simulink model "Projekt_KUS_sim"  (R2013a)
settings: Solver=ode45  SolverMode=SingleTasking  StartTime=0.0  StopTime=1.0  RelTol=1e-3
undefined symbols (not defined in the file): B, Mn, psien, R, T, Un
settings Model: Creator=user  LastModifiedBy=Jarek
settings DataIOCC: SignalLoggingSaveFormat=ModelDataLogs
settings OptimizationCC: BlockReduction=off  BooleanDataType=off
settings DebuggingCC: SaveWithParameterizedLinksMsg=none  SignalResolutionControl=TryResolveAllWithWarning  SolverPrmCheckMsg=none  MultiTaskDSMMsg=warning  MultiTaskCondExecSysMsg=none  StrictBusMsg=None
settings HardwareCC: TargetUnknown=on
settings RTWCC: IncludeERTFirstTime=on

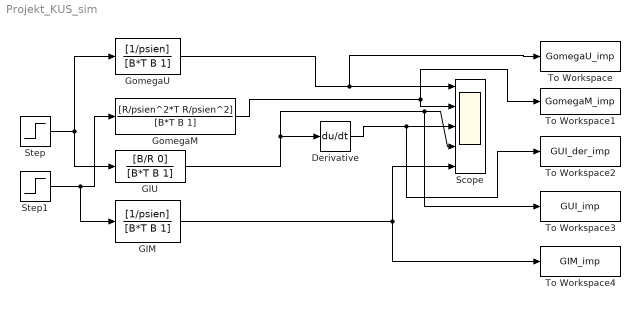
== system Projekt_KUS_sim ==
  Derivative : Derivative
  GIM : TransferFcn  Numerator=[1/psien]  Denominator=[B*T B 1]
  GIU : TransferFcn  Numerator=[B/R 0]  Denominator=[B*T B 1]
  GomegaM : TransferFcn  Numerator=[R/psien^2*T R/psien^2]  Denominator=[B*T B 1]
  GomegaU : TransferFcn  Numerator=[1/psien]  Denominator=[B*T B 1]
  Scope : Scope  NumInputPorts=5
      settings: YMin=-5~-5~-5~-5~-5  YMax=200~20~50~5~5
  Step : Step  Time=0  After=Un  SampleTime=0
  Step1 : Step  Time=0  After=Mn  SampleTime=0
  To Workspace : ToWorkspace  VariableName=GomegaU_imp  SampleTime=-1  SaveFormat=Structure With Time
  To Workspace1 : ToWorkspace  VariableName=GomegaM_imp  SampleTime=-1  SaveFormat=Structure With Time
  To Workspace2 : ToWorkspace  VariableName=GUI_der_imp  SampleTime=-1  SaveFormat=Structure With Time
  To Workspace3 : ToWorkspace  VariableName=GUI_imp  SampleTime=-1  SaveFormat=Structure With Time
  To Workspace4 : ToWorkspace  VariableName=GIM_imp  SampleTime=-1  SaveFormat=Structure With Time
  wires:
  GIU/1 -> To Workspace3/1, Scope/4, Derivative/1
  Derivative/1 -> To Workspace2/1, Scope/3
  GomegaU/1 -> To Workspace/1, Scope/1
  GIM/1 -> Scope/5, To Workspace4/1
  Step1/1 -> GIM/1, GomegaM/1
  Step/1 -> GomegaU/1, GIU/1
  GomegaM/1 -> Scope/2, To Workspace1/1
